simulink model "L1E3"  (R2019b)
settings: Solver=VariableStepAuto  StartTime=0.0  StopTime=100  RelTol=1e-3
model workspace (MAT data in the model file):
  k = Simulink.Parameter
  k.Value = 5.7
  k.DataType = 'auto'
  k.Dimensions = [1 1]
  m = Simulink.Parameter
  m.DataType = 'auto'
  m.Dimensions = [0 0]
  wn = Simulink.Parameter
  wn.Value = 1
  wn.DataType = 'auto'
  wn.Dimensions = [1 1]
  zeta = Simulink.Parameter
  zeta.Value = 5
  zeta.DataType = 'auto'
  zeta.Dimensions = [1 1]
settings Model: Creator=Callum  LastModifiedBy=Callum
settings DataIOCC: ReturnWorkspaceOutputs=off

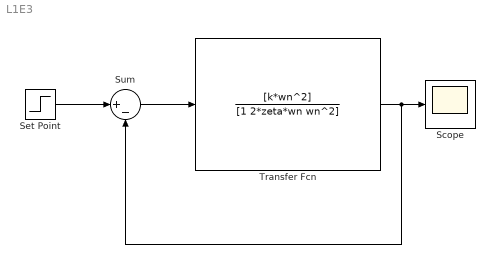
== system L1E3 ==
  Scope : Scope
  Set Point : Step  Time=10  SampleTime=0
  Sum : Sum  Inputs=|+-
  Transfer Fcn : TransferFcn  Numerator=[k*wn^2]  Denominator=[1 2*zeta*wn wn^2]
  wires:
  Set Point/1 -> Sum/1
  Sum/1 -> Transfer Fcn/1
  Transfer Fcn/1 -> Sum/2, Scope/1
